simulink subsystem "kCalculation"  (R2021b)
settings: Solver=VariableStepAuto  StartTime=0.0  StopTime=10.0  RelTol=1e-3
undefined symbols (not defined in the file): kScale
settings Model: Creator=Jiaqi  LastModifiedBy=Jiaqi

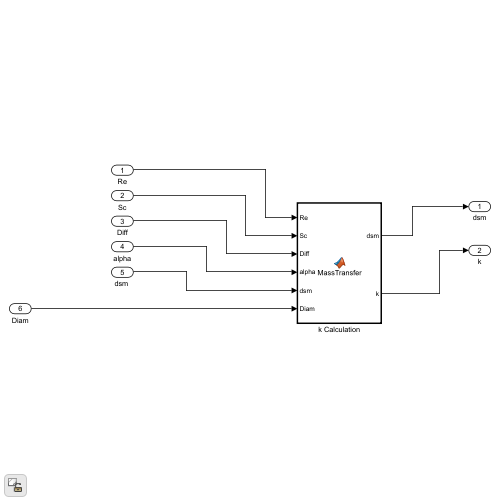
[thumbnail: Simulink's stored preview of the top-level diagram]
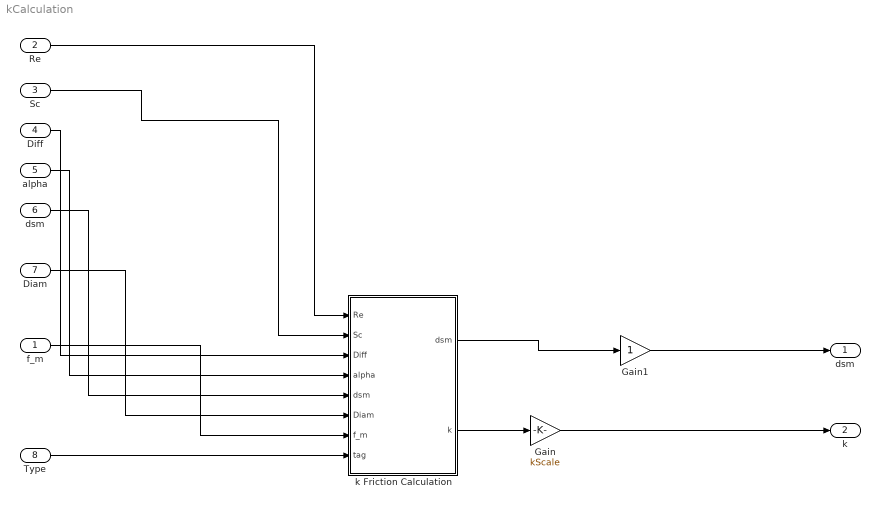
== system kCalculation ==
  f_m : Inport
  Re : Inport  Port=2
  Sc : Inport  Port=3
  Diff : Inport  Port=4
  alpha : Inport  Port=5
  "dsm " : Inport  Port=6
  Diam : Inport  Port=7
  Type : Inport  Port=8
  Gain : Gain  Gain=kScale
  Gain1 : Gain
  k Friction Calculation : MATLAB Function  TreatAsAtomicUnit=on
  dsm : Outport
  k : Outport  Port=2
  wires:
  alpha/1 -> k Friction Calculation/4(alpha)
  Re/1 -> k Friction Calculation/1(Re)
  k Friction Calculation/2(k) -> Gain/1
  Sc/1 -> k Friction Calculation/2(Sc)
  Diff/1 -> k Friction Calculation/3(Diff)
  Diam/1 -> k Friction Calculation/6(Diam)
  "dsm "/1 -> k Friction Calculation/5("dsm ")
  Gain/1 -> k/1
  k Friction Calculation/1(dsm) -> Gain1/1
  Gain1/1 -> dsm/1
  f_m/1 -> k Friction Calculation/7(f_m)
  Type/1 -> k Friction Calculation/8(tag)

== matlab function kCalculation/k Friction Calculation ==
  data: dsm output; Re input; k output; Sc input; Diff input; alpha input; dsm input; Diam input; f_m input; tag input
function [dsm, k] = MassTransfer(Re, Sc, Diff, alpha, dsm, Diam, f_m, tag)
    
    %Simulation regression model. The model by Kress has that weird d/D
    %which is hard to say.
    if strcmp(tag,'upwards')
        Sh = 0.6038*abs(Re)^0.6044*abs(Sc)^0.5;
    elseif strcmp(tag,'downwards')
        Sh = 1.0644*abs(Re)^0.5382*abs(Sc)^0.5;
    elseif isnumeric(tag)
        %Mixed upwards and downwards, tag represent upwards fraction.
        Sh = tag*0.6038*abs(Re)^0.6044*abs(Sc)^0.5 + (1-tag)*1.0644*abs(Re)^0.5382*abs(Sc)^0.5;
    else
        Sh = 0.763*abs(Re)^0.552*abs(Sc)^0.5;
    end
        %Everything else is horizontal.
        Sh_fm = 0.3364*abs(Sc)^0.5*abs(Re)^0.75*abs(f_m)^0.25;
        Sh = max(Sh,Sh_fm);
        k = Sh/Diam*abs(Diff);

end
